simulink model "mytopology7"  (R2015a)
settings: Solver=ode23tb  StartTime=0.0  StopTime=1  MaxStep=0.0001  MinStep=0.00001  RelTol=1e-3
libraries: powerlib x70, simulink x42, powerlib_meascontrol x2
settings Model: CovSFcnEnable=off  Creator=HOME  LastModifiedBy=SELVA
settings DataIOCC: SignalLoggingSaveFormat=ModelDataLogs
settings OptimizationCC: ExpressionDepthLimit=2147483647
settings DebuggingCC: UnderspecifiedInitializationDetection=Classic  MergeDetectMultiDrivingBlocksExec=none  SolverPrmCheckMsg=warning  FcnCallInpInsideContextMsg=UseLocalSettings  StateNameClashWarn=warning
settings GRTTargetCC: CombineOutputUpdateFcns=off  GRTInterface=on

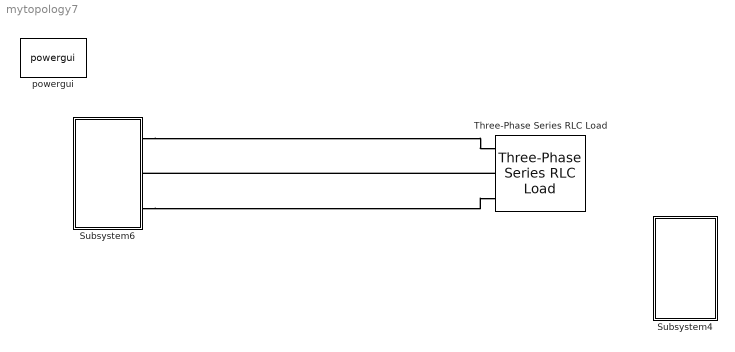
== system mytopology7 ==
  Subsystem4 : Subsystem
  Subsystem6 : Subsystem  mask{m=1, fc=1000, v=230, c1=22000e-6}
      mask prompts: m "Modulation Index"; fc "Switching Frequency"; v "1 Phase Input Voltage"; c1 "DC Link Capacitor"
  Three-Phase Series RLC Load : powerlib/Elements/Three-Phase Series RLC Load  LConnTagsString=A|B|C  Configuration=Y (grounded)  NominalVoltage=400  NominalFrequency=50  ActivePower=4e3  InductivePower=00  CapacitivePower=0  Measurements=None  LoadType=constant Z
  powergui : powerlib/powergui  Priority=1  SimulationMode=Discrete  SolverType=Tustin/Backward Euler (TBE)  SampleTime=50e-6  frequency=60  SPID=off  DisableSnubberDevices=off  DisableRonSwitches=off  DisableVfSwitches=off  SwTol=0  DisplayEquations=off  Interpol=off  methode=off  Ts=100  FunctionMessages=off  echomessages=off  HookPort=off  EnableUseOfTLC=off  x0status=blocks  frequencyindice=0  Pbase=100e6  ErrMax=1e-4  Iterations=50  UnitsV=kV  UnitsW=MW  buscounter=0  RestoreLinks=warning  ResistiveCurrentMeasurement=off  Frange=[0:2:500]  Ylog=off  Xlog=on  ShowGrid=off  save=off  variable=ZData  structure=ScopeData1  ZoomFFT=off  StartTime=0.1  cycles=1  DisplayStyle=1  fundamental=50  FreqAxis=off  MaxFrequency=1000  frequencyindicesteady=1  RmsSteady=1  display=off
  connections:
  Subsystem6/RConn1 -- Three-Phase Series RLC Load/LConn1
  Three-Phase Series RLC Load/LConn2 -- Subsystem6/RConn2
  Subsystem6/RConn3 -- Three-Phase Series RLC Load/LConn3

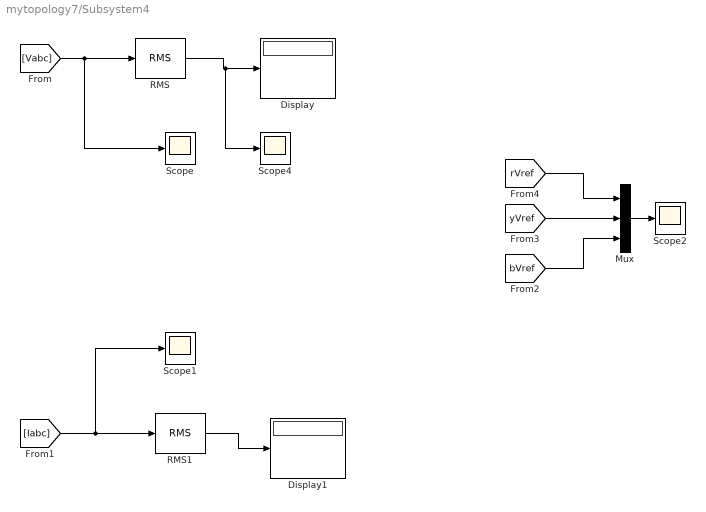
== system mytopology7/Subsystem4 ==
  Display : Display
  Display1 : Display
  Mux : Mux  Inputs=3
  RMS : powerlib_meascontrol/Measurements/RMS  TrueRMS=on  Freq=50  RMSInit=120  Ts=0
  RMS1 : powerlib_meascontrol/Measurements/RMS  TrueRMS=on  Freq=50  RMSInit=120  Ts=0
  Scope{,1..2,4} (4 alike) : Scope
      Scope settings: YMin=-1000  YMax=1000
      Scope1 settings: YMin=-40  YMax=30  SaveName=ScopeData2
      Scope2 settings: YMin=-1  YMax=1  SaveName=ScopeData4
      Scope4 settings: YMin=-600  YMax=600  SaveName=ScopeData3
  wires:
  [Vabc] -> Scope/1, RMS/1
  [Iabc] -> RMS1/1, Scope1/1
  RMS/1 -> Scope4/1, Display/1
  RMS1/1 -> Display1/1
  Mux/1 -> Scope2/1
  [bVref] -> Mux/3
  [rVref] -> Mux/1
  [yVref] -> Mux/2

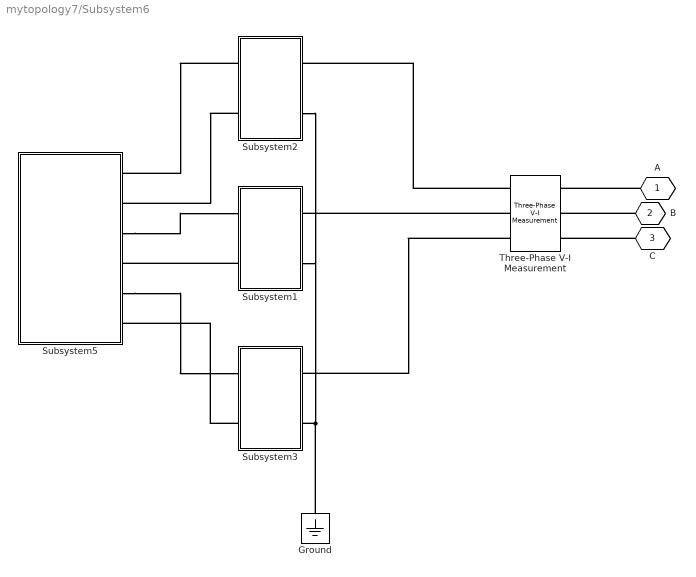
== system mytopology7/Subsystem6 ==
  Ground : powerlib/Elements/Ground  LConnTagsString=a
  Subsystem1 : Subsystem
  Subsystem2 : Subsystem
  Subsystem3 : Subsystem
  Subsystem5 : Subsystem
  Three-Phase V-I Measurement : powerlib/Measurements/Three-Phase V-I Measurement  VoltageMeasurement=phase-to-ground  SetLabelV=on  LabelV=Vabc  Vpu=off  VpuLL=off  CurrentMeasurement=yes  SetLabelI=on  LabelI=Iabc  Ipu=off  Pbase=100e6  Vbase=500e3  OutputType=Complex  PhasorSimulation=off  PSBequivalent=0
  A : PMIOPort  Port=1  Side=Right
  B : PMIOPort  Port=2  Side=Right
  C : PMIOPort  Port=3  Side=Right
  connections:
  Subsystem3/RConn2 -- Ground/LConn1 -- Subsystem2/RConn2 -- Subsystem1/RConn2
  Three-Phase V-I Measurement/LConn3 -- Subsystem3/RConn1
  Three-Phase V-I Measurement/LConn2 -- Subsystem1/RConn1
  Three-Phase V-I Measurement/LConn1 -- Subsystem2/RConn1
  A/RConn1 -- Three-Phase V-I Measurement/RConn1
  B/RConn1 -- Three-Phase V-I Measurement/RConn2
  C/RConn1 -- Three-Phase V-I Measurement/RConn3
  Subsystem2/LConn1 -- Subsystem5/RConn1
  Subsystem2/LConn2 -- Subsystem5/RConn2
  Subsystem5/RConn3 -- Subsystem1/LConn1
  Subsystem1/LConn2 -- Subsystem5/RConn4
  Subsystem5/RConn5 -- Subsystem3/LConn1
  Subsystem3/LConn2 -- Subsystem5/RConn6

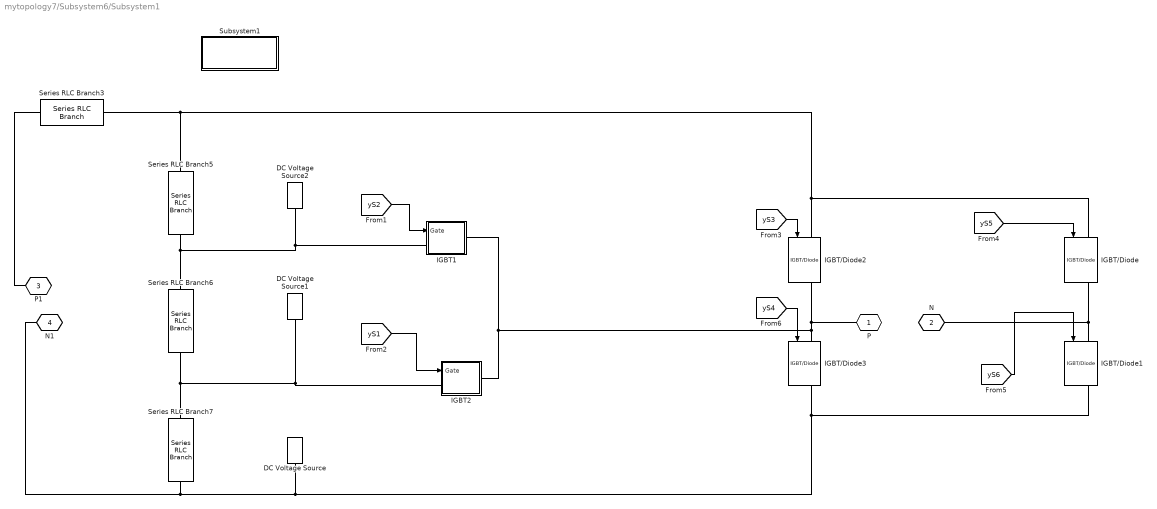
== system mytopology7/Subsystem6/Subsystem1 ==
  DC Voltage Source : powerlib/Electrical Sources/DC Voltage Source  Amplitude=c1  Measurements=None
  DC Voltage Source1 : powerlib/Electrical Sources/DC Voltage Source  Amplitude=c1  Measurements=None
  DC Voltage Source2 : powerlib/Electrical Sources/DC Voltage Source  Amplitude=c1  Measurements=None
  IGBT/Diode{,1..3} (4 alike) : powerlib/Power Electronics/IGBT//Diode  Ron=1e-3  Rs=1e5  Cs=inf  Measurements=on
  IGBT1 : Subsystem
  IGBT2 : Subsystem
  Series RLC Branch3 : powerlib/Elements/Series RLC Branch  LConnTagsString=__new0  RConnTagsString=__new0  BranchType=R  Resistance=0.001  Inductance=1e-3  SetiL0=off  InitialCurrent=0  Capacitance=10e-3  Setx0=off  InitialVoltage=0  Measurements=None
  Series RLC Branch5 : powerlib/Elements/Series RLC Branch  LConnTagsString=__new0  RConnTagsString=__new0  BranchType=C  Resistance=1  Inductance=1e-3  SetiL0=off  InitialCurrent=0  Capacitance=c1  Setx0=off  InitialVoltage=0  Measurements=None
  Series RLC Branch6 : powerlib/Elements/Series RLC Branch  LConnTagsString=__new0  RConnTagsString=__new0  BranchType=C  Resistance=1  Inductance=1e-3  SetiL0=off  InitialCurrent=0  Capacitance=c1  Setx0=off  InitialVoltage=0  Measurements=None
  Series RLC Branch7 : powerlib/Elements/Series RLC Branch  LConnTagsString=__new0  RConnTagsString=__new0  BranchType=C  Resistance=1  Inductance=1e-3  SetiL0=off  InitialCurrent=0  Capacitance=c1  Setx0=off  InitialVoltage=0  Measurements=None
  Subsystem1 : Subsystem
  P : PMIOPort  Port=1  Side=Right
  N : PMIOPort  Port=2  Side=Right
  P1 : PMIOPort  Port=3  Side=Left
  N1 : PMIOPort  Port=4  Side=Left
  wires:
  [yS4] -> IGBT/Diode3/1
  [yS3] -> IGBT/Diode2/1
  [yS6] -> IGBT/Diode1/1
  [yS5] -> IGBT/Diode/1
  [yS1] -> IGBT2/1(Gate)
  [yS2] -> IGBT1/1(Gate)
  connections:
  N/RConn1 -- IGBT/Diode/RConn1 -- IGBT/Diode1/LConn1
  IGBT/Diode1/RConn1 -- IGBT/Diode3/RConn1 -- DC Voltage Source/LConn1 -- Series RLC Branch7/RConn1 -- N1/RConn1
  P1/RConn1 -- Series RLC Branch3/RConn1
  IGBT2/RConn1 -- IGBT1/RConn1 -- IGBT/Diode3/LConn1 -- P/RConn1 -- IGBT/Diode2/RConn1
  IGBT/Diode2/LConn1 -- Series RLC Branch5/LConn1 -- Series RLC Branch3/LConn1 -- IGBT/Diode/LConn1
  IGBT2/LConn1 -- Series RLC Branch6/RConn1 -- Series RLC Branch7/LConn1 -- DC Voltage Source1/LConn1
  IGBT1/LConn1 -- DC Voltage Source2/LConn1 -- Series RLC Branch5/RConn1 -- Series RLC Branch6/LConn1

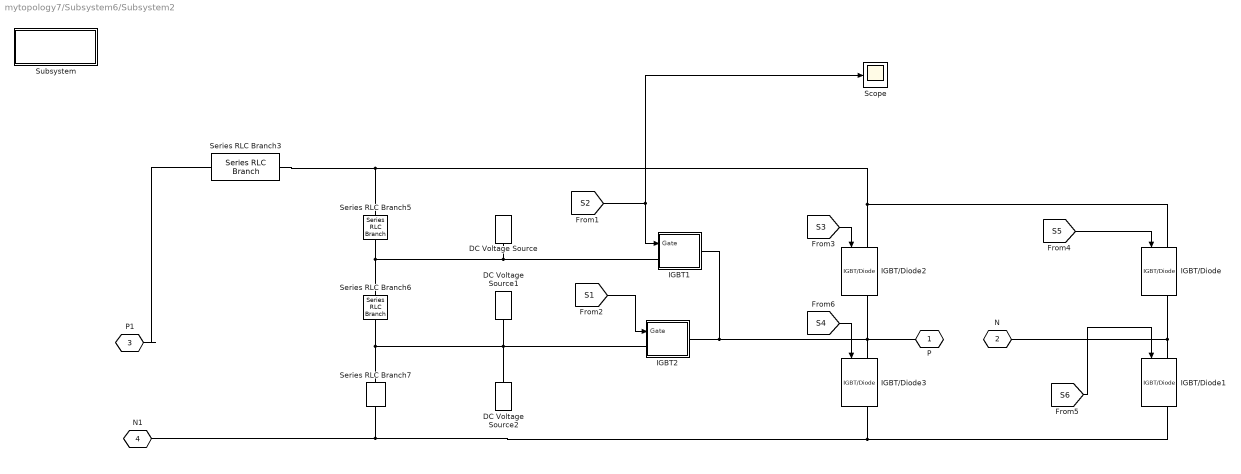
== system mytopology7/Subsystem6/Subsystem2 ==
  DC Voltage Source : powerlib/Electrical Sources/DC Voltage Source  Amplitude=c1  Measurements=None
  DC Voltage Source1 : powerlib/Electrical Sources/DC Voltage Source  Amplitude=c1  Measurements=None
  DC Voltage Source2 : powerlib/Electrical Sources/DC Voltage Source  Amplitude=c1  Measurements=None
  IGBT/Diode{,1..3} (4 alike) : powerlib/Power Electronics/IGBT//Diode  Ron=1e-3  Rs=1e5  Cs=inf  Measurements=on
  IGBT1 : Subsystem
  IGBT2 : Subsystem
  Scope : Scope
  Series RLC Branch3 : powerlib/Elements/Series RLC Branch  LConnTagsString=__new0  RConnTagsString=__new0  BranchType=R  Resistance=0.001  Inductance=1e-3  SetiL0=off  InitialCurrent=0  Capacitance=10e-3  Setx0=off  InitialVoltage=0  Measurements=None
  Series RLC Branch5 : powerlib/Elements/Series RLC Branch  LConnTagsString=__new0  RConnTagsString=__new0  BranchType=C  Resistance=1  Inductance=1e-3  SetiL0=off  InitialCurrent=0  Capacitance=c1  Setx0=off  InitialVoltage=0  Measurements=None
  Series RLC Branch6 : powerlib/Elements/Series RLC Branch  LConnTagsString=__new0  RConnTagsString=__new0  BranchType=C  Resistance=1  Inductance=1e-3  SetiL0=off  InitialCurrent=0  Capacitance=c1  Setx0=off  InitialVoltage=0  Measurements=None
  Series RLC Branch7 : powerlib/Elements/Series RLC Branch  LConnTagsString=__new0  RConnTagsString=__new0  BranchType=C  Resistance=1  Inductance=1e-3  SetiL0=off  InitialCurrent=0  Capacitance=c1  Setx0=off  InitialVoltage=0  Measurements=None
  Subsystem : Subsystem
  P : PMIOPort  Port=1  Side=Right
  N : PMIOPort  Port=2  Side=Right
  P1 : PMIOPort  Port=3  Side=Left
  N1 : PMIOPort  Port=4  Side=Left
  wires:
  [S2] -> IGBT1/1(Gate), Scope/1
  [S1] -> IGBT2/1(Gate)
  [S5] -> IGBT/Diode/1
  [S6] -> IGBT/Diode1/1
  [S3] -> IGBT/Diode2/1
  [S4] -> IGBT/Diode3/1
  connections:
  Series RLC Branch3/LConn1 -- IGBT/Diode/LConn1 -- IGBT/Diode2/LConn1 -- Series RLC Branch5/LConn1
  P/RConn1 -- IGBT1/RConn1 -- IGBT2/RConn1 -- IGBT/Diode3/LConn1 -- IGBT/Diode2/RConn1
  P1/RConn1 -- Series RLC Branch3/RConn1
  IGBT/Diode1/RConn1 -- Series RLC Branch7/RConn1 -- N1/RConn1 -- IGBT/Diode3/RConn1
  IGBT/Diode/RConn1 -- N/RConn1 -- IGBT/Diode1/LConn1
  IGBT1/LConn1 -- Series RLC Branch5/RConn1 -- Series RLC Branch6/LConn1 -- DC Voltage Source/LConn1
  IGBT2/LConn1 -- Series RLC Branch7/LConn1 -- Series RLC Branch6/RConn1 -- DC Voltage Source2/RConn1 -- DC Voltage Source1/LConn1

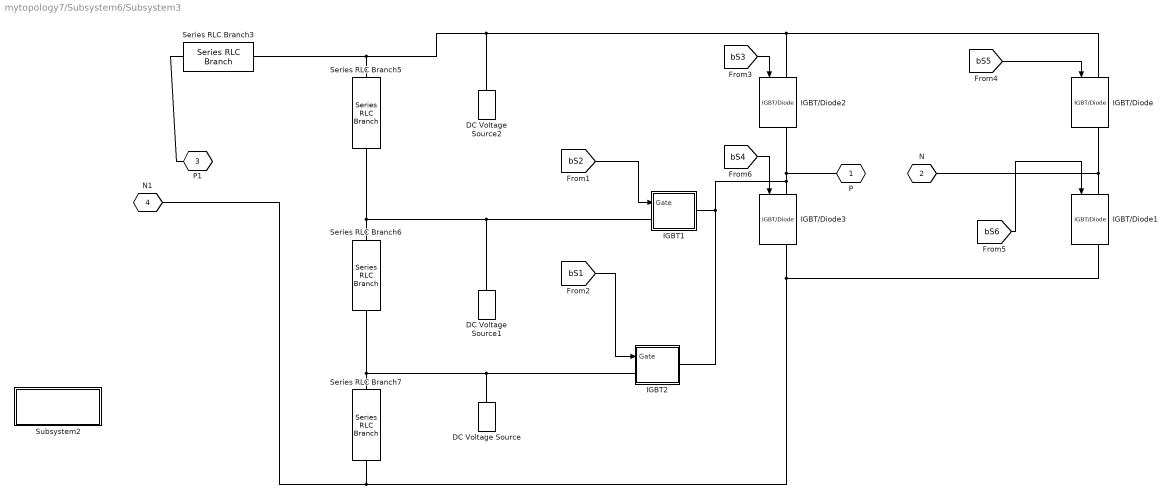
== system mytopology7/Subsystem6/Subsystem3 ==
  DC Voltage Source : powerlib/Electrical Sources/DC Voltage Source  Amplitude=c1  Measurements=None
  DC Voltage Source1 : powerlib/Electrical Sources/DC Voltage Source  Amplitude=c1  Measurements=None
  DC Voltage Source2 : powerlib/Electrical Sources/DC Voltage Source  Amplitude=c1  Measurements=None
  IGBT/Diode{,1..3} (4 alike) : powerlib/Power Electronics/IGBT//Diode  Ron=1e-3  Rs=1e5  Cs=inf  Measurements=on
  IGBT1 : Subsystem
  IGBT2 : Subsystem
  Series RLC Branch3 : powerlib/Elements/Series RLC Branch  LConnTagsString=__new0  RConnTagsString=__new0  BranchType=R  Resistance=0.001  Inductance=1e-3  SetiL0=off  InitialCurrent=0  Capacitance=10e-3  Setx0=off  InitialVoltage=0  Measurements=None
  Series RLC Branch5 : powerlib/Elements/Series RLC Branch  LConnTagsString=__new0  RConnTagsString=__new0  BranchType=C  Resistance=1  Inductance=1e-3  SetiL0=off  InitialCurrent=0  Capacitance=c1  Setx0=off  InitialVoltage=0  Measurements=None
  Series RLC Branch6 : powerlib/Elements/Series RLC Branch  LConnTagsString=__new0  RConnTagsString=__new0  BranchType=C  Resistance=1  Inductance=1e-3  SetiL0=off  InitialCurrent=0  Capacitance=c1  Setx0=off  InitialVoltage=0  Measurements=None
  Series RLC Branch7 : powerlib/Elements/Series RLC Branch  LConnTagsString=__new0  RConnTagsString=__new0  BranchType=C  Resistance=1  Inductance=1e-3  SetiL0=off  InitialCurrent=0  Capacitance=c1  Setx0=off  InitialVoltage=0  Measurements=None
  Subsystem2 : Subsystem
  P : PMIOPort  Port=1  Side=Right
  N : PMIOPort  Port=2  Side=Right
  P1 : PMIOPort  Port=3  Side=Left
  N1 : PMIOPort  Port=4  Side=Left
  wires:
  [bS2] -> IGBT1/1(Gate)
  [bS1] -> IGBT2/1(Gate)
  [bS5] -> IGBT/Diode/1
  [bS6] -> IGBT/Diode1/1
  [bS3] -> IGBT/Diode2/1
  [bS4] -> IGBT/Diode3/1
  connections:
  IGBT/Diode/LConn1 -- Series RLC Branch5/LConn1 -- Series RLC Branch3/LConn1 -- DC Voltage Source2/RConn1 -- IGBT/Diode2/LConn1
  P/RConn1 -- IGBT/Diode2/RConn1 -- IGBT/Diode3/LConn1 -- IGBT1/RConn1 -- IGBT2/RConn1
  Series RLC Branch3/RConn1 -- P1/RConn1
  IGBT/Diode3/RConn1 -- IGBT/Diode1/RConn1 -- Series RLC Branch7/RConn1 -- N1/RConn1
  IGBT/Diode1/LConn1 -- N/RConn1 -- IGBT/Diode/RConn1
  IGBT1/LConn1 -- Series RLC Branch5/RConn1 -- Series RLC Branch6/LConn1 -- DC Voltage Source1/RConn1
  IGBT2/LConn1 -- Series RLC Branch6/RConn1 -- Series RLC Branch7/LConn1 -- DC Voltage Source/RConn1

== system mytopology7/Subsystem6/Subsystem5 ==
  DC Voltage Source : powerlib/Electrical Sources/DC Voltage Source  Amplitude=v*1.414  Measurements=None
  DC Voltage Source1 : powerlib/Electrical Sources/DC Voltage Source  Amplitude=v*1.414  Measurements=None
  DC Voltage Source2 : powerlib/Electrical Sources/DC Voltage Source  Amplitude=v*1.414  Measurements=None
  P1 : PMIOPort  Port=1  Side=Right
  N1 : PMIOPort  Port=2  Side=Right
  P2 : PMIOPort  Port=3  Side=Right
  N2 : PMIOPort  Port=4  Side=Right
  P3 : PMIOPort  Port=5  Side=Right
  N3 : PMIOPort  Port=6  Side=Right
  connections:
  DC Voltage Source/RConn1 -- P1/RConn1
  N1/RConn1 -- DC Voltage Source/LConn1
  DC Voltage Source1/RConn1 -- P2/RConn1
  N2/RConn1 -- DC Voltage Source1/LConn1
  DC Voltage Source2/RConn1 -- P3/RConn1
  N3/RConn1 -- DC Voltage Source2/LConn1

== system mytopology7/Subsystem6/Subsystem1/IGBT1 ==
  Gate : Inport
  Diode{,1..3} (4 alike) : powerlib/Power Electronics/Diode  Ron=0.001  Lon=0  Vf=0.8  IC=0  UseSnubber=off  Rs=500  Cs=250e-9  Measurements=on
  IGBT/Diode : powerlib/Power Electronics/IGBT//Diode  Ron=1e-3  Rs=1e5  Cs=inf  Measurements=on
  C : PMIOPort  Port=1  Side=Left
  E : PMIOPort  Port=2  Side=Right
  wires:
  Gate/1 -> IGBT/Diode/1
  connections:
  Diode/RConn1 -- Diode2/RConn1 -- IGBT/Diode/LConn1
  Diode1/LConn1 -- Diode3/LConn1 -- IGBT/Diode/RConn1
  Diode2/LConn1 -- Diode3/RConn1 -- C/RConn1
  Diode1/RConn1 -- Diode/LConn1 -- E/RConn1

== system mytopology7/Subsystem6/Subsystem1/IGBT2 ==
  Gate : Inport
  Diode{,1..3} (4 alike) : powerlib/Power Electronics/Diode  Ron=0.001  Lon=0  Vf=0.8  IC=0  UseSnubber=off  Rs=500  Cs=250e-9  Measurements=on
  IGBT/Diode : powerlib/Power Electronics/IGBT//Diode  Ron=1e-3  Rs=1e5  Cs=inf  Measurements=on
  C : PMIOPort  Port=1  Side=Left
  E : PMIOPort  Port=2  Side=Right
  wires:
  Gate/1 -> IGBT/Diode/1
  connections:
  E/RConn1 -- Diode/LConn1 -- Diode1/RConn1
  C/RConn1 -- Diode3/RConn1 -- Diode2/LConn1
  IGBT/Diode/RConn1 -- Diode3/LConn1 -- Diode1/LConn1
  IGBT/Diode/LConn1 -- Diode2/RConn1 -- Diode/RConn1

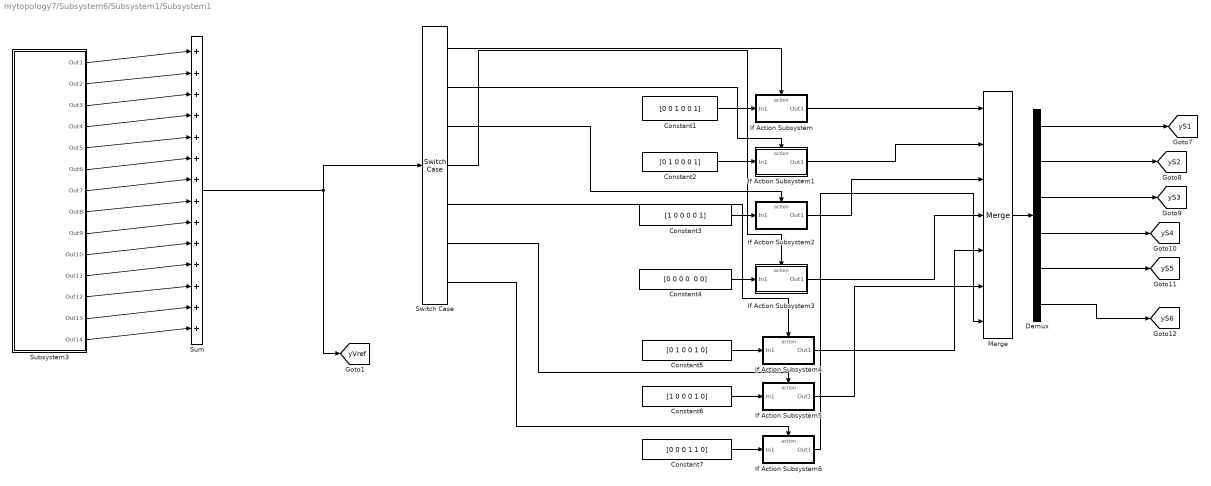
== system mytopology7/Subsystem6/Subsystem1/Subsystem1 ==
  Constant1 : Constant  Value=[0 0 1 0 0 1]
  Constant2 : Constant  Value=[0 1 0 0 0 1]
  Constant3 : Constant  Value=[1 0 0 0 0 1]
  Constant4 : Constant  Value="[0 0 0 0  0 0]"
  Constant5 : Constant  Value=[0 1 0 0 1 0]
  Constant6 : Constant  Value=[1 0 0 0 1 0]
  Constant7 : Constant  Value=[0 0 0 1 1 0]
  Demux : Demux  Outputs=6
  If Action Subsystem : Subsystem  TreatAsAtomicUnit=on
  If Action Subsystem1 : Subsystem  TreatAsAtomicUnit=on
  If Action Subsystem2 : Subsystem  TreatAsAtomicUnit=on
  If Action Subsystem3 : Subsystem  TreatAsAtomicUnit=on
  If Action Subsystem4 : Subsystem  TreatAsAtomicUnit=on
  If Action Subsystem5 : Subsystem  TreatAsAtomicUnit=on
  If Action Subsystem6 : Subsystem  TreatAsAtomicUnit=on
  Merge : Merge  Inputs=7
  Subsystem3 : Subsystem
  Sum : Sum  Inputs=|++++++++++++++
  Switch Case : SwitchCase  CaseConditions="{3 2 1  0 -1 -2 -3}"  ShowDefaultCase=off
  tag scope: yS1=global, yS2=global, yS3=global, yS4=global, yS5=global, yS6=global, yVref=global
  wires:
  Subsystem3/1(Out1) -> Sum/1
  Subsystem3/6(Out6) -> Sum/6
  Subsystem3/7(Out7) -> Sum/7
  Subsystem3/10(Out10) -> Sum/10
  Subsystem3/9(Out9) -> Sum/9
  Subsystem3/8(Out8) -> Sum/8
  Subsystem3/5(Out5) -> Sum/5
  Subsystem3/4(Out4) -> Sum/4
  Subsystem3/2(Out2) -> Sum/2
  Subsystem3/3(Out3) -> Sum/3
  Subsystem3/14(Out14) -> Sum/14
  Subsystem3/12(Out12) -> Sum/12
  Subsystem3/13(Out13) -> Sum/13
  Subsystem3/11(Out11) -> Sum/11
  Constant1/1 -> If Action Subsystem/1(In1)
  Constant2/1 -> If Action Subsystem1/1(In1)
  Constant3/1 -> If Action Subsystem2/1(In1)
  Constant4/1 -> If Action Subsystem3/1(In1)
  Constant5/1 -> If Action Subsystem4/1(In1)
  If Action Subsystem/1(Out1) -> Merge/1
  If Action Subsystem1/1(Out1) -> Merge/2
  If Action Subsystem2/1(Out1) -> Merge/3
  If Action Subsystem3/1(Out1) -> Merge/4
  If Action Subsystem4/1(Out1) -> Merge/5
  Merge/1 -> Demux/1
  Demux/2 -> [yS2]
  Demux/3 -> [yS3]
  Demux/4 -> [yS4]
  Demux/1 -> [yS1]
  Demux/5 -> [yS5]
  Constant6/1 -> If Action Subsystem5/1(In1)
  Constant7/1 -> If Action Subsystem6/1(In1)
  If Action Subsystem6/1(Out1) -> Merge/7
  If Action Subsystem5/1(Out1) -> Merge/6
  Demux/6 -> [yS6]
  Switch Case/1 -> If Action Subsystem/Action
  Switch Case/2 -> If Action Subsystem1/Action
  Switch Case/3 -> If Action Subsystem2/Action
  Switch Case/4 -> If Action Subsystem3/Action
  Switch Case/5 -> If Action Subsystem4/Action
  Switch Case/6 -> If Action Subsystem5/Action
  Switch Case/7 -> If Action Subsystem6/Action
  Sum/1 -> [yVref], Switch Case/1

== system mytopology7/Subsystem6/Subsystem2/IGBT1 ==
  Gate : Inport
  Diode{,1..3} (4 alike) : powerlib/Power Electronics/Diode  Ron=0.001  Lon=0  Vf=0.8  IC=0  UseSnubber=off  Rs=500  Cs=250e-9  Measurements=on
  IGBT/Diode : powerlib/Power Electronics/IGBT//Diode  Ron=1e-3  Rs=1e5  Cs=inf  Measurements=on
  C : PMIOPort  Port=1  Side=Left
  E : PMIOPort  Port=2  Side=Right
  wires:
  Gate/1 -> IGBT/Diode/1
  connections:
  E/RConn1 -- Diode/LConn1 -- Diode1/RConn1
  C/RConn1 -- Diode3/RConn1 -- Diode2/LConn1
  IGBT/Diode/RConn1 -- Diode3/LConn1 -- Diode1/LConn1
  IGBT/Diode/LConn1 -- Diode2/RConn1 -- Diode/RConn1

== system mytopology7/Subsystem6/Subsystem2/IGBT2 ==
  Gate : Inport
  Diode{,1..3} (4 alike) : powerlib/Power Electronics/Diode  Ron=0.001  Lon=0  Vf=0.8  IC=0  UseSnubber=off  Rs=500  Cs=250e-9  Measurements=on
  IGBT/Diode : powerlib/Power Electronics/IGBT//Diode  Ron=1e-3  Rs=1e5  Cs=inf  Measurements=on
  C : PMIOPort  Port=1  Side=Left
  E : PMIOPort  Port=2  Side=Right
  wires:
  Gate/1 -> IGBT/Diode/1
  connections:
  Diode/RConn1 -- Diode2/RConn1 -- IGBT/Diode/LConn1
  Diode1/LConn1 -- Diode3/LConn1 -- IGBT/Diode/RConn1
  Diode2/LConn1 -- Diode3/RConn1 -- C/RConn1
  Diode1/RConn1 -- Diode/LConn1 -- E/RConn1

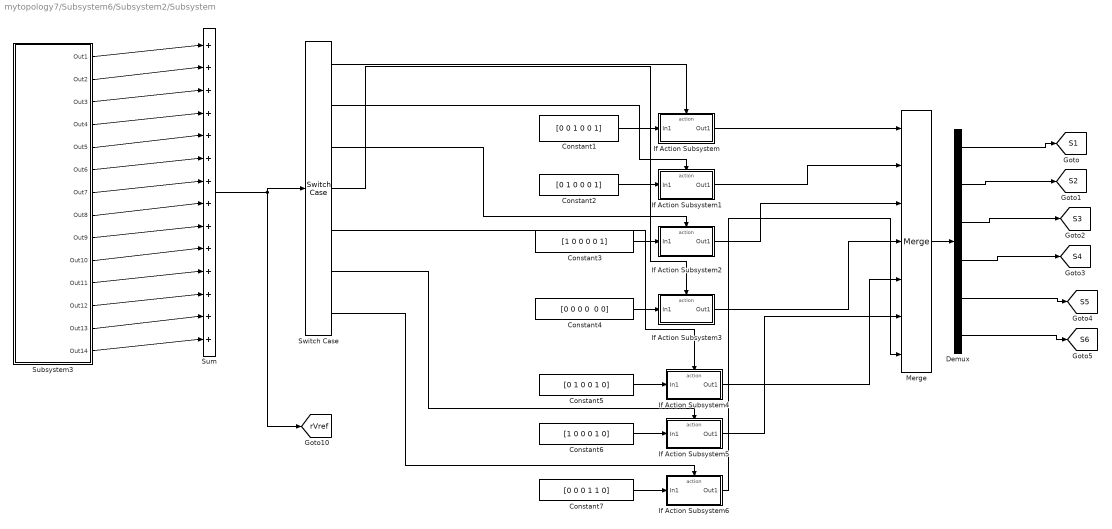
== system mytopology7/Subsystem6/Subsystem2/Subsystem ==
  Constant1 : Constant  Value=[0 0 1 0 0 1]
  Constant2 : Constant  Value=[0 1 0 0 0 1]
  Constant3 : Constant  Value=[1 0 0 0 0 1]
  Constant4 : Constant  Value="[0 0 0 0  0 0]"
  Constant5 : Constant  Value=[0 1 0 0 1 0]
  Constant6 : Constant  Value=[1 0 0 0 1 0]
  Constant7 : Constant  Value=[0 0 0 1 1 0]
  Demux : Demux  Outputs=6
  If Action Subsystem : Subsystem  TreatAsAtomicUnit=on
  If Action Subsystem1 : Subsystem  TreatAsAtomicUnit=on
  If Action Subsystem2 : Subsystem  TreatAsAtomicUnit=on
  If Action Subsystem3 : Subsystem  TreatAsAtomicUnit=on
  If Action Subsystem4 : Subsystem  TreatAsAtomicUnit=on
  If Action Subsystem5 : Subsystem  TreatAsAtomicUnit=on
  If Action Subsystem6 : Subsystem  TreatAsAtomicUnit=on
  Merge : Merge  Inputs=7
  Subsystem3 : Subsystem
  Sum : Sum  Inputs=|++++++++++++++
  Switch Case : SwitchCase  CaseConditions="{3 2 1  0 -1 -2 -3}"  ShowDefaultCase=off
  tag scope: S1=global, S2=global, S3=global, S4=global, S5=global, S6=global, rVref=global
  wires:
  Constant1/1 -> If Action Subsystem/1(In1)
  Constant2/1 -> If Action Subsystem1/1(In1)
  Constant3/1 -> If Action Subsystem2/1(In1)
  Constant4/1 -> If Action Subsystem3/1(In1)
  Constant5/1 -> If Action Subsystem4/1(In1)
  If Action Subsystem/1(Out1) -> Merge/1
  If Action Subsystem1/1(Out1) -> Merge/2
  If Action Subsystem2/1(Out1) -> Merge/3
  If Action Subsystem3/1(Out1) -> Merge/4
  If Action Subsystem4/1(Out1) -> Merge/5
  Merge/1 -> Demux/1
  Demux/2 -> [S2]
  Demux/3 -> [S3]
  Demux/4 -> [S4]
  Demux/1 -> [S1]
  Demux/5 -> [S5]
  Constant6/1 -> If Action Subsystem5/1(In1)
  Constant7/1 -> If Action Subsystem6/1(In1)
  If Action Subsystem6/1(Out1) -> Merge/7
  If Action Subsystem5/1(Out1) -> Merge/6
  Demux/6 -> [S6]
  Switch Case/1 -> If Action Subsystem/Action
  Switch Case/2 -> If Action Subsystem1/Action
  Switch Case/3 -> If Action Subsystem2/Action
  Switch Case/4 -> If Action Subsystem3/Action
  Switch Case/5 -> If Action Subsystem4/Action
  Switch Case/6 -> If Action Subsystem5/Action
  Switch Case/7 -> If Action Subsystem6/Action
  Subsystem3/1(Out1) -> Sum/1
  Subsystem3/6(Out6) -> Sum/6
  Subsystem3/7(Out7) -> Sum/7
  Subsystem3/10(Out10) -> Sum/10
  Subsystem3/9(Out9) -> Sum/9
  Subsystem3/8(Out8) -> Sum/8
  Subsystem3/5(Out5) -> Sum/5
  Subsystem3/4(Out4) -> Sum/4
  Subsystem3/2(Out2) -> Sum/2
  Subsystem3/3(Out3) -> Sum/3
  Subsystem3/14(Out14) -> Sum/14
  Subsystem3/12(Out12) -> Sum/12
  Subsystem3/13(Out13) -> Sum/13
  Subsystem3/11(Out11) -> Sum/11
  Sum/1 -> Switch Case/1, [rVref]

== system mytopology7/Subsystem6/Subsystem3/IGBT1 ==
  Gate : Inport
  Diode{,1..3} (4 alike) : powerlib/Power Electronics/Diode  Ron=0.001  Lon=0  Vf=0.8  IC=0  UseSnubber=off  Rs=500  Cs=250e-9  Measurements=on
  IGBT/Diode : powerlib/Power Electronics/IGBT//Diode  Ron=1e-3  Rs=1e5  Cs=inf  Measurements=on
  C : PMIOPort  Port=1  Side=Left
  E : PMIOPort  Port=2  Side=Right
  wires:
  Gate/1 -> IGBT/Diode/1
  connections:
  E/RConn1 -- Diode/LConn1 -- Diode1/RConn1
  C/RConn1 -- Diode3/RConn1 -- Diode2/LConn1
  IGBT/Diode/RConn1 -- Diode3/LConn1 -- Diode1/LConn1
  IGBT/Diode/LConn1 -- Diode2/RConn1 -- Diode/RConn1

== system mytopology7/Subsystem6/Subsystem3/IGBT2 ==
  Gate : Inport
  Diode{,1..3} (4 alike) : powerlib/Power Electronics/Diode  Ron=0.001  Lon=0  Vf=0.8  IC=0  UseSnubber=off  Rs=500  Cs=250e-9  Measurements=on
  IGBT/Diode : powerlib/Power Electronics/IGBT//Diode  Ron=1e-3  Rs=1e5  Cs=inf  Measurements=on
  C : PMIOPort  Port=1  Side=Left
  E : PMIOPort  Port=2  Side=Right
  wires:
  Gate/1 -> IGBT/Diode/1
  connections:
  Diode/RConn1 -- Diode2/RConn1 -- IGBT/Diode/LConn1
  Diode1/LConn1 -- Diode3/LConn1 -- IGBT/Diode/RConn1
  Diode2/LConn1 -- Diode3/RConn1 -- C/RConn1
  Diode1/RConn1 -- Diode/LConn1 -- E/RConn1

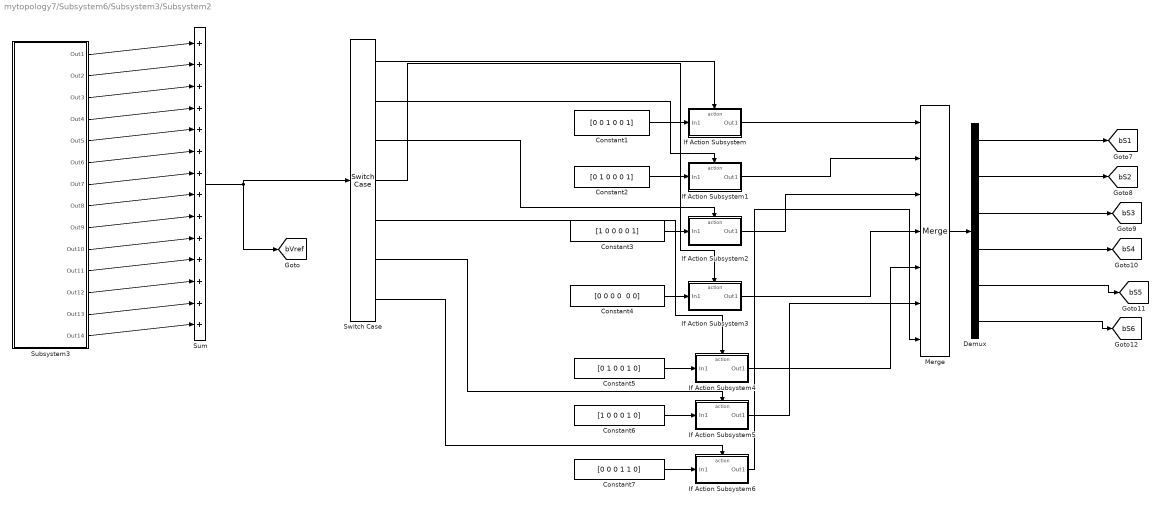
== system mytopology7/Subsystem6/Subsystem3/Subsystem2 ==
  Constant1 : Constant  Value=[0 0 1 0 0 1]
  Constant2 : Constant  Value=[0 1 0 0 0 1]
  Constant3 : Constant  Value=[1 0 0 0 0 1]
  Constant4 : Constant  Value="[0 0 0 0  0 0]"
  Constant5 : Constant  Value=[0 1 0 0 1 0]
  Constant6 : Constant  Value=[1 0 0 0 1 0]
  Constant7 : Constant  Value=[0 0 0 1 1 0]
  Demux : Demux  Outputs=6
  If Action Subsystem : Subsystem  TreatAsAtomicUnit=on
  If Action Subsystem1 : Subsystem  TreatAsAtomicUnit=on
  If Action Subsystem2 : Subsystem  TreatAsAtomicUnit=on
  If Action Subsystem3 : Subsystem  TreatAsAtomicUnit=on
  If Action Subsystem4 : Subsystem  TreatAsAtomicUnit=on
  If Action Subsystem5 : Subsystem  TreatAsAtomicUnit=on
  If Action Subsystem6 : Subsystem  TreatAsAtomicUnit=on
  Merge : Merge  Inputs=7
  Subsystem3 : Subsystem
  Sum : Sum  Inputs=|++++++++++++++
  Switch Case : SwitchCase  CaseConditions="{3 2 1  0 -1 -2 -3}"  ShowDefaultCase=off
  tag scope: bS1=global, bS2=global, bS3=global, bS4=global, bS5=global, bS6=global, bVref=global
  wires:
  Subsystem3/1(Out1) -> Sum/1
  Subsystem3/6(Out6) -> Sum/6
  Subsystem3/7(Out7) -> Sum/7
  Subsystem3/10(Out10) -> Sum/10
  Subsystem3/9(Out9) -> Sum/9
  Subsystem3/8(Out8) -> Sum/8
  Subsystem3/5(Out5) -> Sum/5
  Subsystem3/4(Out4) -> Sum/4
  Subsystem3/2(Out2) -> Sum/2
  Subsystem3/3(Out3) -> Sum/3
  Subsystem3/14(Out14) -> Sum/14
  Subsystem3/12(Out12) -> Sum/12
  Subsystem3/13(Out13) -> Sum/13
  Subsystem3/11(Out11) -> Sum/11
  Constant1/1 -> If Action Subsystem/1(In1)
  Constant2/1 -> If Action Subsystem1/1(In1)
  Constant3/1 -> If Action Subsystem2/1(In1)
  Constant4/1 -> If Action Subsystem3/1(In1)
  Constant5/1 -> If Action Subsystem4/1(In1)
  If Action Subsystem/1(Out1) -> Merge/1
  If Action Subsystem1/1(Out1) -> Merge/2
  If Action Subsystem2/1(Out1) -> Merge/3
  If Action Subsystem3/1(Out1) -> Merge/4
  If Action Subsystem4/1(Out1) -> Merge/5
  Merge/1 -> Demux/1
  Demux/2 -> [bS2]
  Demux/3 -> [bS3]
  Demux/4 -> [bS4]
  Demux/1 -> [bS1]
  Demux/5 -> [bS5]
  Constant6/1 -> If Action Subsystem5/1(In1)
  Constant7/1 -> If Action Subsystem6/1(In1)
  If Action Subsystem6/1(Out1) -> Merge/7
  If Action Subsystem5/1(Out1) -> Merge/6
  Demux/6 -> [bS6]
  Switch Case/1 -> If Action Subsystem/Action
  Switch Case/2 -> If Action Subsystem1/Action
  Switch Case/3 -> If Action Subsystem2/Action
  Switch Case/4 -> If Action Subsystem3/Action
  Switch Case/5 -> If Action Subsystem4/Action
  Switch Case/6 -> If Action Subsystem5/Action
  Switch Case/7 -> If Action Subsystem6/Action
  Sum/1 -> [bVref], Switch Case/1

== system mytopology7/Subsystem6/Subsystem1/Subsystem1/If Action Subsystem ==
  In1 : Inport
  Action Port : ActionPort  ActionType=case
  Out1 : Outport
  wires:
  In1/1 -> Out1/1

== system mytopology7/Subsystem6/Subsystem1/Subsystem1/If Action Subsystem1 ==
  In1 : Inport
  Action Port : ActionPort  ActionType=case
  Out1 : Outport
  wires:
  In1/1 -> Out1/1

== system mytopology7/Subsystem6/Subsystem1/Subsystem1/If Action Subsystem2 ==
  In1 : Inport
  Action Port : ActionPort  ActionType=case
  Out1 : Outport
  wires:
  In1/1 -> Out1/1

== system mytopology7/Subsystem6/Subsystem1/Subsystem1/If Action Subsystem3 ==
  In1 : Inport
  Action Port : ActionPort  ActionType=case
  Out1 : Outport
  wires:
  In1/1 -> Out1/1

== system mytopology7/Subsystem6/Subsystem1/Subsystem1/If Action Subsystem4 ==
  In1 : Inport
  Action Port : ActionPort  ActionType=case
  Out1 : Outport
  wires:
  In1/1 -> Out1/1

== system mytopology7/Subsystem6/Subsystem1/Subsystem1/If Action Subsystem5 ==
  In1 : Inport
  Action Port : ActionPort  ActionType=case
  Out1 : Outport
  wires:
  In1/1 -> Out1/1

== system mytopology7/Subsystem6/Subsystem1/Subsystem1/If Action Subsystem6 ==
  In1 : Inport
  Action Port : ActionPort  ActionType=case
  Out1 : Outport
  wires:
  In1/1 -> Out1/1

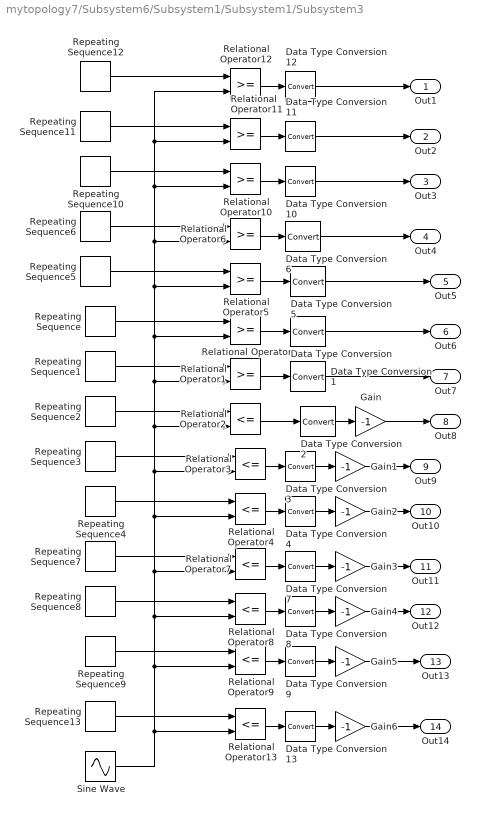
== system mytopology7/Subsystem6/Subsystem1/Subsystem1/Subsystem3 ==
  Data Type Conversion{,1..13} (14 alike) : DataTypeConversion
  Gain{,1..6} (7 alike) : Gain  Gain=-1
  Relational Operator{,1,5..6,10..12} (7 alike) : RelationalOperator  OutDataTypeStr=boolean
  Relational Operator{2..4,7..9,13} (7 alike) : RelationalOperator  Operator=<=  OutDataTypeStr=boolean
  Repeating Sequence : simulink/Sources/Repeating Sequence  rep_seq_t="[0 (1/fc)/2  (1/fc)]"  rep_seq_y=[1 2 1]
  Repeating Sequence1 : simulink/Sources/Repeating Sequence  rep_seq_t="[0 (1/fc)/2  (1/fc)]"  rep_seq_y=[0 1 0]
  Repeating Sequence10 : simulink/Sources/Repeating Sequence  rep_seq_t="[0 (1/fc)/2  (1/fc)]"  rep_seq_y=[4 5 4]
  Repeating Sequence11 : simulink/Sources/Repeating Sequence  rep_seq_t="[0 (1/fc)/2  (1/fc)]"  rep_seq_y=[5 6 5]
  Repeating Sequence12 : simulink/Sources/Repeating Sequence  rep_seq_t="[0 (1/fc)/2  (1/fc)]"  rep_seq_y=[6 7 6]
  Repeating Sequence13 : simulink/Sources/Repeating Sequence  rep_seq_t="[0 (1/fc)/2  (1/fc)]"  rep_seq_y=[-7 -6 -7]
  Repeating Sequence2 : simulink/Sources/Repeating Sequence  rep_seq_t="[0 (1/fc)/2  (1/fc)]"  rep_seq_y=[-1 0 -1]
  Repeating Sequence3 : simulink/Sources/Repeating Sequence  rep_seq_t="[0 (1/fc)/2  (1/fc)]"  rep_seq_y=[-2 -1 -2]
  Repeating Sequence4 : simulink/Sources/Repeating Sequence  rep_seq_t="[0 (1/fc)/2  (1/fc)]"  rep_seq_y=[-3 -2 -3]
  Repeating Sequence5 : simulink/Sources/Repeating Sequence  rep_seq_t="[0 (1/fc)/2  (1/fc)]"  rep_seq_y=[2 3 2]
  Repeating Sequence6 : simulink/Sources/Repeating Sequence  rep_seq_t="[0 (1/fc)/2  (1/fc)]"  rep_seq_y=[3 4 3]
  Repeating Sequence7 : simulink/Sources/Repeating Sequence  rep_seq_t="[0 (1/fc)/2  (1/fc)]"  rep_seq_y=[-4 -3 -4]
  Repeating Sequence8 : simulink/Sources/Repeating Sequence  rep_seq_t="[0 (1/fc)/2  (1/fc)]"  rep_seq_y=[-5 -4 -5]
  Repeating Sequence9 : simulink/Sources/Repeating Sequence  rep_seq_t="[0 (1/fc)/2  (1/fc)]"  rep_seq_y=[-6 -5 -6]
  Sine Wave : Sin  Amplitude=3*m  Frequency=2*pi*50  Phase=2*pi/3  SampleTime=0
  Out1 : Outport
  Out2 : Outport  Port=2
  Out3 : Outport  Port=3
  Out4 : Outport  Port=4
  Out5 : Outport  Port=5
  Out6 : Outport  Port=6
  Out7 : Outport  Port=7
  Out8 : Outport  Port=8
  Out9 : Outport  Port=9
  Out10 : Outport  Port=10
  Out11 : Outport  Port=11
  Out12 : Outport  Port=12
  Out13 : Outport  Port=13
  Out14 : Outport  Port=14
  wires:
  Relational Operator/1 -> Data Type Conversion/1
  Relational Operator1/1 -> Data Type Conversion1/1
  Repeating Sequence/1 -> Relational Operator/1
  Repeating Sequence1/1 -> Relational Operator1/1
  Repeating Sequence2/1 -> Relational Operator2/1
  Repeating Sequence3/1 -> Relational Operator3/1
  Relational Operator2/1 -> Data Type Conversion2/1
  Relational Operator3/1 -> Data Type Conversion3/1
  Data Type Conversion2/1 -> Gain/1
  Data Type Conversion3/1 -> Gain1/1
  Repeating Sequence4/1 -> Relational Operator4/1
  Relational Operator4/1 -> Data Type Conversion4/1
  Data Type Conversion4/1 -> Gain2/1
  Relational Operator5/1 -> Data Type Conversion5/1
  Repeating Sequence5/1 -> Relational Operator5/1
  Relational Operator6/1 -> Data Type Conversion6/1
  Repeating Sequence6/1 -> Relational Operator6/1
  Repeating Sequence7/1 -> Relational Operator7/1
  Relational Operator7/1 -> Data Type Conversion7/1
  Data Type Conversion7/1 -> Gain3/1
  Repeating Sequence8/1 -> Relational Operator8/1
  Relational Operator8/1 -> Data Type Conversion8/1
  Data Type Conversion8/1 -> Gain4/1
  Repeating Sequence9/1 -> Relational Operator9/1
  Relational Operator9/1 -> Data Type Conversion9/1
  Data Type Conversion9/1 -> Gain5/1
  Repeating Sequence10/1 -> Relational Operator10/1
  Relational Operator10/1 -> Data Type Conversion10/1
  Sine Wave/1 -> Relational Operator13/2, Relational Operator9/2, Relational Operator8/2, Relational Operator7/2, Relational Operator4/2, Relational Operator3/2, Relational Operator2/2, Relational Operator1/2, Relational Operator/2, Relational Operator5/2, Relational Operator6/2, Relational Operator10/2, Relational Operator11/2, Relational Operator12/2
  Repeating Sequence11/1 -> Relational Operator11/1
  Relational Operator11/1 -> Data Type Conversion11/1
  Relational Operator12/1 -> Data Type Conversion12/1
  Repeating Sequence12/1 -> Relational Operator12/1
  Repeating Sequence13/1 -> Relational Operator13/1
  Relational Operator13/1 -> Data Type Conversion13/1
  Data Type Conversion13/1 -> Gain6/1
  Data Type Conversion12/1 -> Out1/1
  Data Type Conversion11/1 -> Out2/1
  Data Type Conversion10/1 -> Out3/1
  Data Type Conversion6/1 -> Out4/1
  Data Type Conversion5/1 -> Out5/1
  Data Type Conversion/1 -> Out6/1
  Data Type Conversion1/1 -> Out7/1
  Gain/1 -> Out8/1
  Gain1/1 -> Out9/1
  Gain2/1 -> Out10/1
  Gain3/1 -> Out11/1
  Gain4/1 -> Out12/1
  Gain5/1 -> Out13/1
  Gain6/1 -> Out14/1

== system mytopology7/Subsystem6/Subsystem2/Subsystem/If Action Subsystem ==
  In1 : Inport
  Action Port : ActionPort  ActionType=case
  Out1 : Outport
  wires:
  In1/1 -> Out1/1

== system mytopology7/Subsystem6/Subsystem2/Subsystem/If Action Subsystem1 ==
  In1 : Inport
  Action Port : ActionPort  ActionType=case
  Out1 : Outport
  wires:
  In1/1 -> Out1/1

== system mytopology7/Subsystem6/Subsystem2/Subsystem/If Action Subsystem2 ==
  In1 : Inport
  Action Port : ActionPort  ActionType=case
  Out1 : Outport
  wires:
  In1/1 -> Out1/1

== system mytopology7/Subsystem6/Subsystem2/Subsystem/If Action Subsystem3 ==
  In1 : Inport
  Action Port : ActionPort  ActionType=case
  Out1 : Outport
  wires:
  In1/1 -> Out1/1

== system mytopology7/Subsystem6/Subsystem2/Subsystem/If Action Subsystem4 ==
  In1 : Inport
  Action Port : ActionPort  ActionType=case
  Out1 : Outport
  wires:
  In1/1 -> Out1/1

== system mytopology7/Subsystem6/Subsystem2/Subsystem/If Action Subsystem5 ==
  In1 : Inport
  Action Port : ActionPort  ActionType=case
  Out1 : Outport
  wires:
  In1/1 -> Out1/1

== system mytopology7/Subsystem6/Subsystem2/Subsystem/If Action Subsystem6 ==
  In1 : Inport
  Action Port : ActionPort  ActionType=case
  Out1 : Outport
  wires:
  In1/1 -> Out1/1

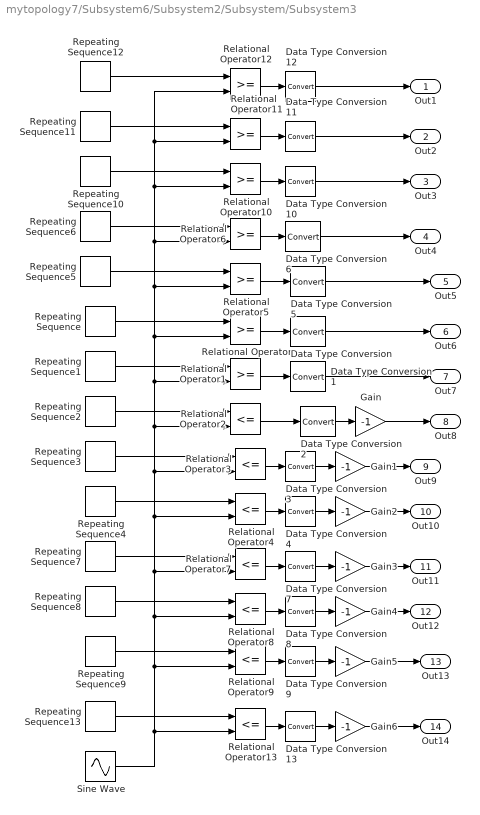
== system mytopology7/Subsystem6/Subsystem2/Subsystem/Subsystem3 ==
  Data Type Conversion{,1..13} (14 alike) : DataTypeConversion
  Gain{,1..6} (7 alike) : Gain  Gain=-1
  Relational Operator{,1,5..6,10..12} (7 alike) : RelationalOperator  OutDataTypeStr=boolean
  Relational Operator{2..4,7..9,13} (7 alike) : RelationalOperator  Operator=<=  OutDataTypeStr=boolean
  Repeating Sequence : simulink/Sources/Repeating Sequence  rep_seq_t="[0 (1/fc)/2  (1/fc)]"  rep_seq_y=[1 2 1]
  Repeating Sequence1 : simulink/Sources/Repeating Sequence  rep_seq_t="[0 (1/fc)/2  (1/fc)]"  rep_seq_y=[0 1 0]
  Repeating Sequence10 : simulink/Sources/Repeating Sequence  rep_seq_t="[0 (1/fc)/2  (1/fc)]"  rep_seq_y=[4 5 4]
  Repeating Sequence11 : simulink/Sources/Repeating Sequence  rep_seq_t="[0 (1/fc)/2  (1/fc)]"  rep_seq_y=[5 6 5]
  Repeating Sequence12 : simulink/Sources/Repeating Sequence  rep_seq_t="[0 (1/fc)/2  (1/fc)]"  rep_seq_y=[6 7 6]
  Repeating Sequence13 : simulink/Sources/Repeating Sequence  rep_seq_t="[0 (1/fc)/2  (1/fc)]"  rep_seq_y=[-7 -6 -7]
  Repeating Sequence2 : simulink/Sources/Repeating Sequence  rep_seq_t="[0 (1/fc)/2  (1/fc)]"  rep_seq_y=[-1 0 -1]
  Repeating Sequence3 : simulink/Sources/Repeating Sequence  rep_seq_t="[0 (1/fc)/2  (1/fc)]"  rep_seq_y=[-2 -1 -2]
  Repeating Sequence4 : simulink/Sources/Repeating Sequence  rep_seq_t="[0 (1/fc)/2  (1/fc)]"  rep_seq_y=[-3 -2 -3]
  Repeating Sequence5 : simulink/Sources/Repeating Sequence  rep_seq_t="[0 (1/fc)/2  (1/fc)]"  rep_seq_y=[2 3 2]
  Repeating Sequence6 : simulink/Sources/Repeating Sequence  rep_seq_t="[0 (1/fc)/2  (1/fc)]"  rep_seq_y=[3 4 3]
  Repeating Sequence7 : simulink/Sources/Repeating Sequence  rep_seq_t="[0 (1/fc)/2  (1/fc)]"  rep_seq_y=[-4 -3 -4]
  Repeating Sequence8 : simulink/Sources/Repeating Sequence  rep_seq_t="[0 (1/fc)/2  (1/fc)]"  rep_seq_y=[-5 -4 -5]
  Repeating Sequence9 : simulink/Sources/Repeating Sequence  rep_seq_t="[0 (1/fc)/2  (1/fc)]"  rep_seq_y=[-6 -5 -6]
  Sine Wave : Sin  Amplitude=3*m  Frequency=2*pi*50  SampleTime=0
  Out1 : Outport
  Out2 : Outport  Port=2
  Out3 : Outport  Port=3
  Out4 : Outport  Port=4
  Out5 : Outport  Port=5
  Out6 : Outport  Port=6
  Out7 : Outport  Port=7
  Out8 : Outport  Port=8
  Out9 : Outport  Port=9
  Out10 : Outport  Port=10
  Out11 : Outport  Port=11
  Out12 : Outport  Port=12
  Out13 : Outport  Port=13
  Out14 : Outport  Port=14
  wires:
  Relational Operator/1 -> Data Type Conversion/1
  Relational Operator1/1 -> Data Type Conversion1/1
  Repeating Sequence/1 -> Relational Operator/1
  Repeating Sequence1/1 -> Relational Operator1/1
  Repeating Sequence2/1 -> Relational Operator2/1
  Repeating Sequence3/1 -> Relational Operator3/1
  Relational Operator2/1 -> Data Type Conversion2/1
  Relational Operator3/1 -> Data Type Conversion3/1
  Data Type Conversion2/1 -> Gain/1
  Data Type Conversion3/1 -> Gain1/1
  Repeating Sequence4/1 -> Relational Operator4/1
  Relational Operator4/1 -> Data Type Conversion4/1
  Data Type Conversion4/1 -> Gain2/1
  Relational Operator5/1 -> Data Type Conversion5/1
  Repeating Sequence5/1 -> Relational Operator5/1
  Relational Operator6/1 -> Data Type Conversion6/1
  Repeating Sequence6/1 -> Relational Operator6/1
  Repeating Sequence7/1 -> Relational Operator7/1
  Relational Operator7/1 -> Data Type Conversion7/1
  Data Type Conversion7/1 -> Gain3/1
  Repeating Sequence8/1 -> Relational Operator8/1
  Relational Operator8/1 -> Data Type Conversion8/1
  Data Type Conversion8/1 -> Gain4/1
  Repeating Sequence9/1 -> Relational Operator9/1
  Relational Operator9/1 -> Data Type Conversion9/1
  Data Type Conversion9/1 -> Gain5/1
  Repeating Sequence10/1 -> Relational Operator10/1
  Relational Operator10/1 -> Data Type Conversion10/1
  Sine Wave/1 -> Relational Operator13/2, Relational Operator9/2, Relational Operator8/2, Relational Operator7/2, Relational Operator4/2, Relational Operator3/2, Relational Operator2/2, Relational Operator1/2, Relational Operator/2, Relational Operator5/2, Relational Operator6/2, Relational Operator10/2, Relational Operator11/2, Relational Operator12/2
  Repeating Sequence11/1 -> Relational Operator11/1
  Relational Operator11/1 -> Data Type Conversion11/1
  Relational Operator12/1 -> Data Type Conversion12/1
  Repeating Sequence12/1 -> Relational Operator12/1
  Repeating Sequence13/1 -> Relational Operator13/1
  Relational Operator13/1 -> Data Type Conversion13/1
  Data Type Conversion13/1 -> Gain6/1
  Data Type Conversion12/1 -> Out1/1
  Data Type Conversion11/1 -> Out2/1
  Data Type Conversion10/1 -> Out3/1
  Data Type Conversion6/1 -> Out4/1
  Data Type Conversion5/1 -> Out5/1
  Data Type Conversion/1 -> Out6/1
  Data Type Conversion1/1 -> Out7/1
  Gain/1 -> Out8/1
  Gain1/1 -> Out9/1
  Gain2/1 -> Out10/1
  Gain3/1 -> Out11/1
  Gain4/1 -> Out12/1
  Gain5/1 -> Out13/1
  Gain6/1 -> Out14/1

== system mytopology7/Subsystem6/Subsystem3/Subsystem2/If Action Subsystem ==
  In1 : Inport
  Action Port : ActionPort  ActionType=case
  Out1 : Outport
  wires:
  In1/1 -> Out1/1

== system mytopology7/Subsystem6/Subsystem3/Subsystem2/If Action Subsystem1 ==
  In1 : Inport
  Action Port : ActionPort  ActionType=case
  Out1 : Outport
  wires:
  In1/1 -> Out1/1

== system mytopology7/Subsystem6/Subsystem3/Subsystem2/If Action Subsystem2 ==
  In1 : Inport
  Action Port : ActionPort  ActionType=case
  Out1 : Outport
  wires:
  In1/1 -> Out1/1

== system mytopology7/Subsystem6/Subsystem3/Subsystem2/If Action Subsystem3 ==
  In1 : Inport
  Action Port : ActionPort  ActionType=case
  Out1 : Outport
  wires:
  In1/1 -> Out1/1

== system mytopology7/Subsystem6/Subsystem3/Subsystem2/If Action Subsystem4 ==
  In1 : Inport
  Action Port : ActionPort  ActionType=case
  Out1 : Outport
  wires:
  In1/1 -> Out1/1

== system mytopology7/Subsystem6/Subsystem3/Subsystem2/If Action Subsystem5 ==
  In1 : Inport
  Action Port : ActionPort  ActionType=case
  Out1 : Outport
  wires:
  In1/1 -> Out1/1

== system mytopology7/Subsystem6/Subsystem3/Subsystem2/If Action Subsystem6 ==
  In1 : Inport
  Action Port : ActionPort  ActionType=case
  Out1 : Outport
  wires:
  In1/1 -> Out1/1

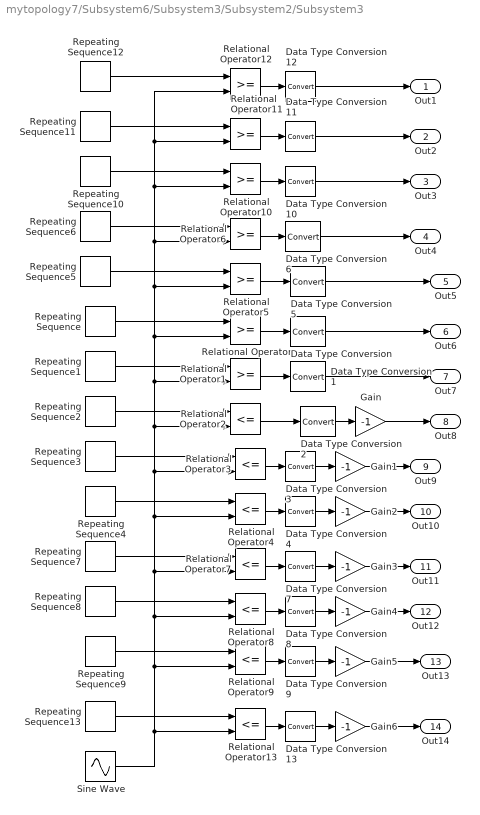
== system mytopology7/Subsystem6/Subsystem3/Subsystem2/Subsystem3 ==
  Data Type Conversion{,1..13} (14 alike) : DataTypeConversion
  Gain{,1..6} (7 alike) : Gain  Gain=-1
  Relational Operator{,1,5..6,10..12} (7 alike) : RelationalOperator  OutDataTypeStr=boolean
  Relational Operator{2..4,7..9,13} (7 alike) : RelationalOperator  Operator=<=  OutDataTypeStr=boolean
  Repeating Sequence : simulink/Sources/Repeating Sequence  rep_seq_t="[0 (1/fc)/2  (1/fc)]"  rep_seq_y=[1 2 1]
  Repeating Sequence1 : simulink/Sources/Repeating Sequence  rep_seq_t="[0 (1/fc)/2  (1/fc)]"  rep_seq_y=[0 1 0]
  Repeating Sequence10 : simulink/Sources/Repeating Sequence  rep_seq_t="[0 (1/fc)/2  (1/fc)]"  rep_seq_y=[4 5 4]
  Repeating Sequence11 : simulink/Sources/Repeating Sequence  rep_seq_t="[0 (1/fc)/2  (1/fc)]"  rep_seq_y=[5 6 5]
  Repeating Sequence12 : simulink/Sources/Repeating Sequence  rep_seq_t="[0 (1/fc)/2  (1/fc)]"  rep_seq_y=[6 7 6]
  Repeating Sequence13 : simulink/Sources/Repeating Sequence  rep_seq_t="[0 (1/fc)/2  (1/fc)]"  rep_seq_y=[-7 -6 -7]
  Repeating Sequence2 : simulink/Sources/Repeating Sequence  rep_seq_t="[0 (1/fc)/2  (1/fc)]"  rep_seq_y=[-1 0 -1]
  Repeating Sequence3 : simulink/Sources/Repeating Sequence  rep_seq_t="[0 (1/fc)/2  (1/fc)]"  rep_seq_y=[-2 -1 -2]
  Repeating Sequence4 : simulink/Sources/Repeating Sequence  rep_seq_t="[0 (1/fc)/2  (1/fc)]"  rep_seq_y=[-3 -2 -3]
  Repeating Sequence5 : simulink/Sources/Repeating Sequence  rep_seq_t="[0 (1/fc)/2  (1/fc)]"  rep_seq_y=[2 3 2]
  Repeating Sequence6 : simulink/Sources/Repeating Sequence  rep_seq_t="[0 (1/fc)/2  (1/fc)]"  rep_seq_y=[3 4 3]
  Repeating Sequence7 : simulink/Sources/Repeating Sequence  rep_seq_t="[0 (1/fc)/2  (1/fc)]"  rep_seq_y=[-4 -3 -4]
  Repeating Sequence8 : simulink/Sources/Repeating Sequence  rep_seq_t="[0 (1/fc)/2  (1/fc)]"  rep_seq_y=[-5 -4 -5]
  Repeating Sequence9 : simulink/Sources/Repeating Sequence  rep_seq_t="[0 (1/fc)/2  (1/fc)]"  rep_seq_y=[-6 -5 -6]
  Sine Wave : Sin  Amplitude=3*m  Frequency=2*pi*50  Phase=-2*pi/3  SampleTime=0
  Out1 : Outport
  Out2 : Outport  Port=2
  Out3 : Outport  Port=3
  Out4 : Outport  Port=4
  Out5 : Outport  Port=5
  Out6 : Outport  Port=6
  Out7 : Outport  Port=7
  Out8 : Outport  Port=8
  Out9 : Outport  Port=9
  Out10 : Outport  Port=10
  Out11 : Outport  Port=11
  Out12 : Outport  Port=12
  Out13 : Outport  Port=13
  Out14 : Outport  Port=14
  wires:
  Relational Operator/1 -> Data Type Conversion/1
  Relational Operator1/1 -> Data Type Conversion1/1
  Repeating Sequence/1 -> Relational Operator/1
  Repeating Sequence1/1 -> Relational Operator1/1
  Repeating Sequence2/1 -> Relational Operator2/1
  Repeating Sequence3/1 -> Relational Operator3/1
  Relational Operator2/1 -> Data Type Conversion2/1
  Relational Operator3/1 -> Data Type Conversion3/1
  Data Type Conversion2/1 -> Gain/1
  Data Type Conversion3/1 -> Gain1/1
  Repeating Sequence4/1 -> Relational Operator4/1
  Relational Operator4/1 -> Data Type Conversion4/1
  Data Type Conversion4/1 -> Gain2/1
  Relational Operator5/1 -> Data Type Conversion5/1
  Repeating Sequence5/1 -> Relational Operator5/1
  Relational Operator6/1 -> Data Type Conversion6/1
  Repeating Sequence6/1 -> Relational Operator6/1
  Repeating Sequence7/1 -> Relational Operator7/1
  Relational Operator7/1 -> Data Type Conversion7/1
  Data Type Conversion7/1 -> Gain3/1
  Repeating Sequence8/1 -> Relational Operator8/1
  Relational Operator8/1 -> Data Type Conversion8/1
  Data Type Conversion8/1 -> Gain4/1
  Repeating Sequence9/1 -> Relational Operator9/1
  Relational Operator9/1 -> Data Type Conversion9/1
  Data Type Conversion9/1 -> Gain5/1
  Repeating Sequence10/1 -> Relational Operator10/1
  Relational Operator10/1 -> Data Type Conversion10/1
  Sine Wave/1 -> Relational Operator13/2, Relational Operator9/2, Relational Operator8/2, Relational Operator7/2, Relational Operator4/2, Relational Operator3/2, Relational Operator2/2, Relational Operator1/2, Relational Operator/2, Relational Operator5/2, Relational Operator6/2, Relational Operator10/2, Relational Operator11/2, Relational Operator12/2
  Repeating Sequence11/1 -> Relational Operator11/1
  Relational Operator11/1 -> Data Type Conversion11/1
  Relational Operator12/1 -> Data Type Conversion12/1
  Repeating Sequence12/1 -> Relational Operator12/1
  Repeating Sequence13/1 -> Relational Operator13/1
  Relational Operator13/1 -> Data Type Conversion13/1
  Data Type Conversion13/1 -> Gain6/1
  Data Type Conversion12/1 -> Out1/1
  Data Type Conversion11/1 -> Out2/1
  Data Type Conversion10/1 -> Out3/1
  Data Type Conversion6/1 -> Out4/1
  Data Type Conversion5/1 -> Out5/1
  Data Type Conversion/1 -> Out6/1
  Data Type Conversion1/1 -> Out7/1
  Gain/1 -> Out8/1
  Gain1/1 -> Out9/1
  Gain2/1 -> Out10/1
  Gain3/1 -> Out11/1
  Gain4/1 -> Out12/1
  Gain5/1 -> Out13/1
  Gain6/1 -> Out14/1
